simulink model "Motor"  (R2021a)
settings: Solver=VariableStepAuto  StartTime=0.0  StopTime=20.0  RelTol=1e-3
libraries: simulink x1
settings Model: Creator=Emily  LastModifiedBy=Emily

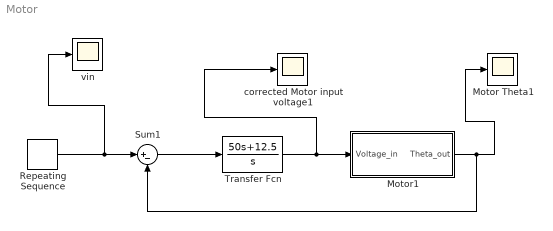
== system Motor ==
  Motor Theta1 : Scope
  Motor1 : Subsystem
  Repeating Sequence : simulink/Sources/Repeating Sequence  rep_seq_t=[0 5 5.01 10 10.01 15 15.01 20]  rep_seq_y=[0 0 2 2 2 2 2 2]
  Sum1 : Sum  Inputs=|+-
  Transfer Fcn : TransferFcn  Numerator=[50 12.5]  Denominator=[1 0]
  corrected Motor input voltage1 : Scope
  vin : Scope
  wires:
  Motor1/1(Theta_out) -> Motor Theta1/1, Sum1/2
  Repeating Sequence/1 -> vin/1, Sum1/1
  Sum1/1 -> Transfer Fcn/1
  Transfer Fcn/1 -> corrected Motor input voltage1/1, Motor1/1(Voltage_in)

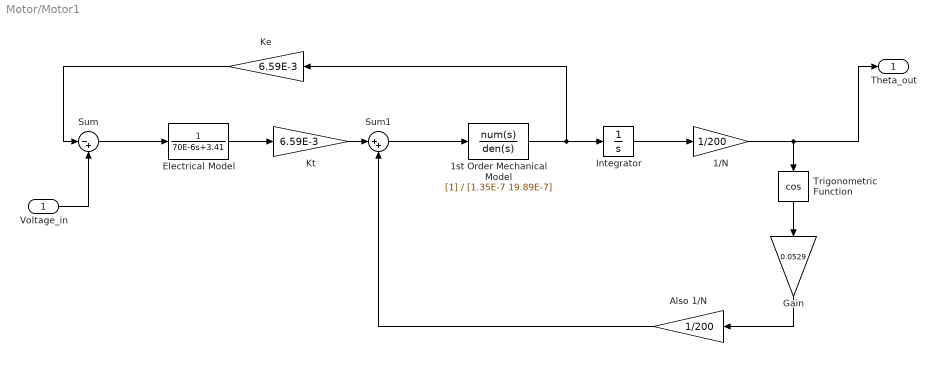
== system Motor/Motor1 ==
  Voltage_in : Inport
  1/N : Gain  Gain=1/200
  1st Order Mechanical Model : TransferFcn  Denominator=[1.35E-7 19.89E-7]
  Also 1/N : Gain  Gain=1/200
  Electrical Model : TransferFcn  Denominator=[70E-6 3.41]
  Gain : Gain  Gain=0.0529
  Integrator : Integrator
  Ke : Gain  Gain=6.59E-3
  Kt : Gain  Gain=6.59E-3
  Sum : Sum  Inputs=|-+
  Sum1 : Sum  Inputs=|++
  Trigonometric Function : Trigonometry  Operator=cos
  Theta_out : Outport
  wires:
  Ke/1 -> Sum/1
  1/N/1 -> Trigonometric Function/1, Theta_out/1
  Electrical Model/1 -> Kt/1
  1st Order Mechanical Model/1 -> Ke/1, Integrator/1
  Integrator/1 -> 1/N/1
  Also 1/N/1 -> Sum1/2
  Sum1/1 -> 1st Order Mechanical Model/1
  Kt/1 -> Sum1/1
  Sum/1 -> Electrical Model/1
  Trigonometric Function/1 -> Gain/1
  Gain/1 -> Also 1/N/1
  Voltage_in/1 -> Sum/2
